simulink model "SMC_ex2"  (R2021a)
settings: Solver=VariableStepAuto  StartTime=0.0  StopTime=10.0  RelTol=1e-3
values from neighbouring files (symbols this model uses):
  a = ksi * ksi * 0.25 * 2    (= 2)    [phase_portrait2.m]    (also in phase_portrait_ex2.m = 8; plot_ex1.m = 8; smc_ex2.m)
  c = 10    [phase_portrait_ex2.m]    (also in plot_ex1.m; smc_ex2.m = -0.732050807569)
  init_conds = zeros(length(angles), 2)    [phase_portrait_ex2.m]    (also in smc_ex2.m = [2, 5])
  ksi = 2    [phase_portrait2.m]    (also in smc_ex2.m)
settings Model: Creator=root  LastModifiedBy=root

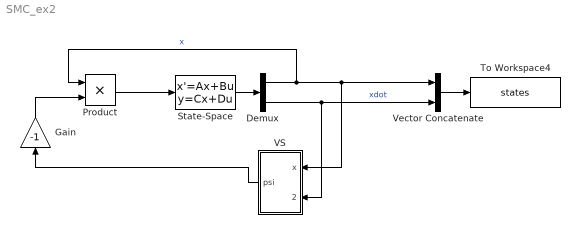
== system SMC_ex2 ==
  Demux : Demux  Outputs=2
  Gain : Gain  Gain=-1
  Product : Product
  State-Space : StateSpace  A=[0 1; 0 ksi]  B=[0; 1]  C=eye(2)  D=zeros(2, 1)  InitialCondition=init_conds
  To Workspace4 : ToWorkspace  VariableName=states  SaveFormat=Timeseries  SampleTime=0.0001
  VS : Subsystem
  Vector Concatenate : Concatenate
  wires:
  Demux/2 -> Vector Concatenate/2, VS/2(xdot)  "xdot"
  Vector Concatenate/1 -> To Workspace4/1
  Demux/1 -> Product/1, Vector Concatenate/1, VS/1(x)  "x"
  VS/1(psi) -> Gain/1
  State-Space/1 -> Demux/1
  Product/1 -> State-Space/1
  Gain/1 -> Product/2

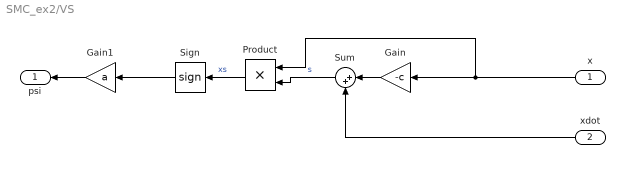
== system SMC_ex2/VS ==
  x : Inport
  xdot : Inport  Port=2
  Gain : Gain  Gain=-c
  Gain1 : Gain  Gain=a
  Product : Product
  Sign : Signum
  Sum : Sum  Inputs=|++
  psi : Outport
  wires:
  Sign/1 -> Gain1/1
  Gain/1 -> Sum/1
  x/1 -> Product/1, Gain/1
  Sum/1 -> Product/2  "s"
  xdot/1 -> Sum/2
  Gain1/1 -> psi/1
  Product/1 -> Sign/1  "xs"
